simulink model "Super1"  (Simulink 8.7)
settings: Solver=ode45  StartTime=0.0  StopTime=10.0  RelTol=1e-3
settings Model: Creator=scaife  LastModifiedBy=bourbouh  ExtModeAutoUpdateStatusClock=off
settings DataIOCC: SignalLoggingSaveFormat=ModelDataLogs  SignalLoggingName=sigsOut
settings DebuggingCC: SaveWithParameterizedLinksMsg=none  SignalResolutionControl=TryResolveAllWithWarning  MultiTaskDSMMsg=warning  MultiTaskCondExecSysMsg=none
settings HardwareCC: TargetUnknown=on
settings SFSimCC: SimParseCustomCode=off
settings GRTTargetCC: GeneratePreprocessorConditionals=Use local settings  CombineOutputUpdateFcns=off  GRTInterface=on

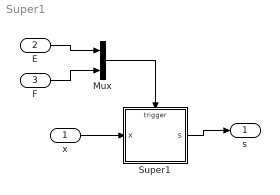
== system Super1 ==
  x : Inport
  E : Inport  Port=2
  F : Inport  Port=3
  Mux : Mux  Inputs=2
  Super1 : Stateflow chart  TreatAsAtomicUnit=on
  s : Outport
  wires:
  x/1 -> Super1/1(x)
  F/1 -> Mux/2
  E/1 -> Mux/1
  Mux/1 -> Super1/Trigger
  Super1/1(s) -> s/1

== stateflow chart Super1 ==
  state A
    en : s = 1;
  state B
    en : s = 5;
  state C
    state C1
      en : s = 3;
    state C2
      en : s = 4;
    (default) -> C1
    C2 -> C1 [order 2] : F
    C1 -> C2 [order 2] : F
  state D
    en : s = 2;
  (default) -> A
  C1 -> B [order 1] : E
  (junction 16) -> C1 [order 1] : [x==0]
  A -> (junction 16) : E
  (junction 16) -> D [order 2] : [x<>0]
  B -> C2 : E
  D -> A : F
  (junction 17) -> A [order 2] : [x==0]
  C2 -> (junction 17) [order 1] : E[x<2]
  (junction 17) -> D [order 1] : [x<>0]
  data: x input uint8; s output uint8
  events: E input EITHER_EDGE_EVENT; F input EITHER_EDGE_EVENT
